simulink model "PID"  (R2024b)
settings: Solver=VariableStepAuto  StartTime=0.0  StopTime=200  FixedStep=1e-3  RelTol=1e-3
undefined symbols (not defined in the file): Orientation, Position
libraries: robotlib x3, simulink_extras x3, sharedutil x2
settings Model: SimulationMode=accelerator  Creator=cdsouza  LastModifiedBy=조홍민
settings SolverCC: ZeroCrossAlgorithm=Adaptive  AlgebraicLoopSolver=TrustRegion
settings DataIOCC: ReturnWorkspaceOutputs=off
settings OptimizationCC: EnhancedBackFolding=on  PassReuseOutputArgsAs=Individual arguments  ZeroExternalMemoryAtStartup=off  ZeroInternalMemoryAtStartup=off  MaxStackSize=64  OptimizeBlockOrder=speed  DifferentSizesBufferReuse=on  EfficientTunableParamExpr=on
settings DebuggingCC: IgnoredZcDiagnostic=none  ParameterTunabilityLossMsg=error  UnconnectedInputMsg=warning  UnconnectedOutputMsg=warning  UnconnectedLineMsg=warning  ArithmeticOperatorsInVariantConditions=warning
settings HardwareCC: ProdBitPerPointer=32  ProdBitPerSizeT=32  ProdBitPerPtrDiffT=32  ProdLargestAtomicFloat=None  ProdIntDivRoundTo=Undefined  ProdEndianess=Unspecified  ProdWordSize=32  ProdHWDeviceType=Generic->Unspecified (assume 32-bit Generic)
settings ModelReferenceCC: EnableRefExpFcnMdlSchedulingChecks=on
settings SFSimCC: MATLABDynamicMemAlloc=off  CustomCodeUndefinedFunction=UseInterfaceOnly
settings RTWCC: Description=Embedded Coder  SystemTargetFile=ert.tlc  HardwareBoard=Robot Operating System (ROS)  TLCOptions="-aInlineSetEventsForThisBaseRateFcn=TLC_FALSE -aSuppressMultiTaskScheduler=TLC_FALSE  -aRateBasedStepFcn=0"  TemplateMakefile=ert_default_tmf  Toolchain=Catkin  TargetLang=C++  GPUComputeCapability=3.5
settings CodeAppCC: ForceParamTrailComments=on  IgnoreCustomStorageClasses=off  OperatorAnnotations=on  SimulinkDataObjDesc=on  SFDataObjDesc=on  InsertBlockDesc=on
settings ERTTargetCC: InlinedParameterPlacement=Hierarchical  DynamicArrayContainerType=coder::array

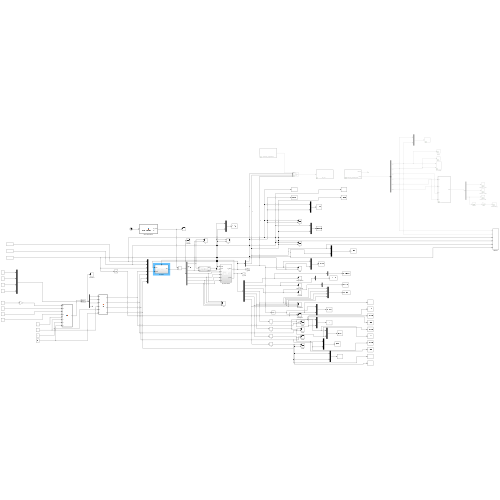
[thumbnail: Simulink's stored preview of the top-level diagram]
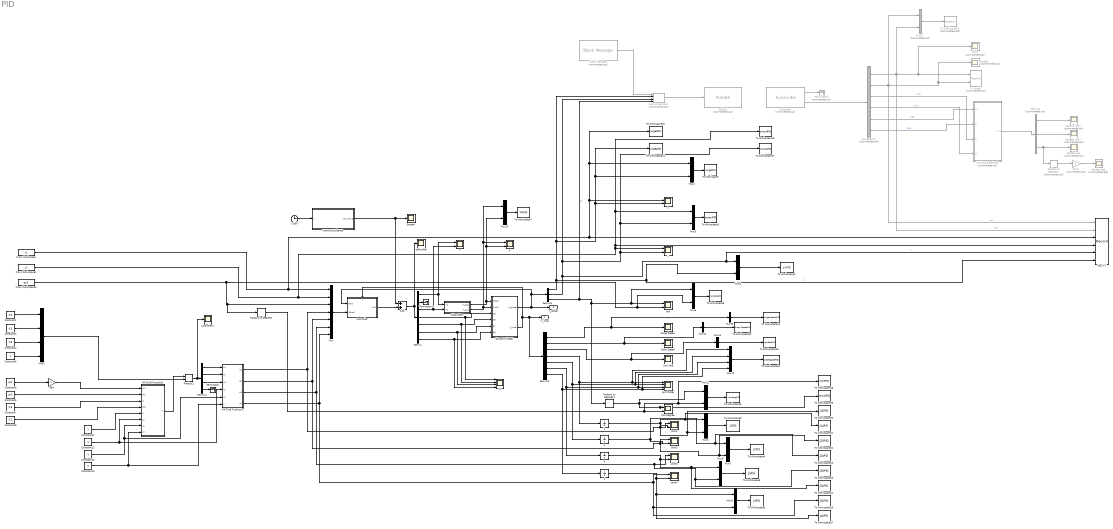
== system PID ==
  {1..4} (4 alike) : Integrator
  Add : Sum
  Blank Message : robotlib/Blank Message  Commented=on  messageClass=Message  entityType=geometry_msgs/Pose  messageType=geometry_msgs/Pose  SampleTime=inf  legacyBusStruct=off
  Bus Assignment : BusAssignment  Commented=on  AssignedSignals=Position.X,Position.Y,Orientation.W
  Bus Selector : BusSelector  Commented=on  OutputSignals=Pose.Position.X,Pose.Position.Y,Pose.Orientation.X,Pose.Orientation.Y,Pose.Orientation.Z,Pose.Orientation.W
  Clock : Clock
  Constant10 : Constant  Value=0
  Constant{5,11..13} (4 alike) : Constant
  Constant2 : Constant  Value=0.5
  Constant3 : Constant  Value=0.3
  Constant4 : Constant  Value=0.8
  Constant6 : Constant  Value=pi/2
  Constant7 : Constant  Value=0.8
  Constant8 : Constant  Value=0.1
  Constant9 : Constant  Value=pi/2
  Controller : Subsystem
      settings: PortSchema="{\"entries\":[{\"content\":{\"sides\":[{\"content\":{\"connectorIds\":[\"In1\",\"In2\"]},\"type\":\"ConnectorPlacement.EquallySpacedRectSide\",\"uuid\":\"f517b411-9821-46d6-bcef-391f15feb496\"},{\"content\":{\"connectorIds\":[\"Out1\"],\"side\":\"RIGHT\"},\"type\":\"ConnectorPlacement.EquallySpacedRectSide\",\"uuid\":\"a797da20-53d3-4f53-a227-0b692005ff54\"},{\"content\":{\"connectorIds\":[\"In3\"],\"side\":\"TOP\"},\"type\":\"ConnectorPlacement.EquallySpacedRectSide\",\"uuid\":\"903174f2-a3c8-433f-ada5-9a38ae3ff1a6\"}]},\"type\":\"ConnectorPlacement.EquallySpacedConnector\",\"uuid\":\"4f0bdd0a-4061-45a8-b959-2bbfa8de12fe\"}],\"packageUris\":[\"http://schema.mathworks.com/mf0/Connector/R2020b\"],\"version\":\"1.0\"}"
  Demux : Demux  Outputs=7
  Demux1 : Demux
  Demux2 : Demux  Outputs=3
  Demux3 : Demux  Outputs=7
  Demux4 : Demux  Commented=on  Outputs=3
  Dynamic Model : Subsystem
  FT : Scope  NumInputPorts=4
  From Workspace : FromWorkspace  VariableName=x1  SampleTime=-1
  From Workspace1 : FromWorkspace  VariableName=y1  SampleTime=-1
  From Workspace2 : FromWorkspace  VariableName=psi1  SampleTime=-1
  Gain : Gain  Gain=-1
  Gain1 : Gain  Commented=on  Gain=-1
  Gazebo Deg : Scope  Commented=on
  Gazebo Yaw : Scope  Commented=on
  Gazebo Yaw1 : Scope  Commented=on
  Gazebo Yaw2 : Scope  Commented=on
  Joint Rates : Scope  NumInputPorts=4
  Joint{1..4} (4 alike) : Scope  NumInputPorts=2
  MATLAB Function1 : MATLAB Function  TreatAsAtomicUnit=on
  MATLAB Function2 : MATLAB Function  TreatAsAtomicUnit=on
  MATLAB Function4 : MATLAB Function  Commented=on  TreatAsAtomicUnit=on
  Mux : Mux  Inputs=7
  Mux1 : Mux
  Mux{2..11} (10 alike) : Mux  Inputs=2
  Mux12 : Mux
  Mux13 : Mux  Inputs=1
  Mux14 : Mux  Inputs=1
  Mux15 : Mux  Inputs=1
  Mux17 : Mux  Commented=on  Inputs=2
  N : Scope  NumInputPorts=2
  NED-XY : Record  FileSettingsInternal="{\"entries\":[{\"content\":{\"excelSettings\":{\"content\":{},\"type\":\"Streamout.ExcelSettings\"}},\"type\":\"Streamout.FileSettingStorage\",\"uuid\":\"\"}],\"packageUris\":[\"http:\\/\\/schema.mathworks.com\\/mf0\\/streamout_blocks\\/R2020a\"],\"version\":\"1.0\"}"  Layout=[1 1]  SignalsInternal="{\"entries\":[{\"content\":{\"signals\":[{\"content\":{\"blockPath\":[],\"dimensions\":[1],\"domain\":\"\",\"lineColor\":\"#a2142f\",\"plots\":[ 1 ],\"port\":1,\"signalID\":1,\"signalName\":\"<Y>\"},\"type\":\"RecordBlkView.Signal\",\"uuid\":\"\"},{\"content\":{\"blockPath\":[],\"dimensions\":[1],\"domain\":\"\",\"lineColor\":\"#139fff\",\"plots\":[ 1 ],\"port\":2,\"signalID\":2,\"signalName\":\"<X>\"},\"type\":\"RecordBlkView.Signal\",\"uuid\":\"\"},{\"content\":{\"blockPath\":[],\"dimensions\":[1],\"domain\":\"\",\"lineColor\":\"#ff6929\",\"plots\":[ 1 ],\"port\":3,\"signalID\":3,\"signalName\":\"From\\nWorkspace\"},\"type\":\"RecordBlkView.Signal\",\"uuid\":\"\"},{\"content\":{\"blockPath\":[],\"dimensions\":[1],\"domain\":\"\",\"lineColor\":\"#b746ff\",\"plots\":[ 1 ],\"port\":4,\"signalID\":4,\"signalName\":\"From\\nWorkspace1\"},\"type\":\"RecordBlkView.Signal\",\"uuid\":\"\"},{\"content\":{\"blockPath\":[],\"dimensions\":[1],\"domain\":\"\",\"lineColor\":\"#139fff\",\"plots\":[ 1 ],\"port\":5,\"signalID\":5,\"signalName\":\"Y\"},\"type\":\"RecordBlkView.Signal\",\"uuid\":\"\"},{\"content\":{\"blockPath\":[],\"dimensions\":[1],\"domain\":\"\",\"lineColor\":\"#ff6929\",\"plots\":[ 1 ],\"port\":6,\"signalID\":6,\"signalName\":\"X\"},\"type\":\"RecordBlkView.Signal\",\"uuid\":\"\"}]},\"type\":\"RecordBlkView.InputSignals\",\"uuid\":\"\"}],\"packageUris\":[\"http:\\/\\/schema.mathworks.com\\/mf0\\/streamout_blocks\\/R2020a\"],\"version\":\"1.0\"}"  VisualizationBindings="{\"xyplotplugin\":{\"info\":[{\"series\":[{\"bindingParametersList\":[{\"parameter\":\"X-Axis\",\"signalID\":1,\"signalName\":\"<Y>\"},{\"parameter\":\"Y-Axis\",\"signalID\":2,\"signalName\":\"<X>\"}],\"seriesID\":0},{\"bindingParametersList\":[{\"parameter\":\"X-Axis\",\"signalID\":4,\"signalName\":\"From\\nWorkspace1\"},{\"parameter\":\"Y-Axis\",\"signalID\":3,\"signalName\":\"From\\nWorkspace\"}],\"seriesID\":1},{\"bindingParametersList\":[{\"parameter\":\"X-Axis\",\"signalID\":5,\"signalName\":\"Y\"},{\"parameter\":\"Y-Axis\",\"signalID\":6,\"signalName\":\"X\"}],\"seriesID\":2}],\"subplotID\":1}]}}"  CompatibilityTag=XY  st=-1
  Product2 : Product  Multiplication=Matrix(*)
  Publish : robotlib/Publish  Commented=on  topicSource=Specify your own  topic=/to_ros  messageType=geometry_msgs/Pose  legacyBusStruct=off  messageQueueLength=1
  Radians to Degrees : simulink_extras/Transformations/Radians to Degrees
  Radians to Degrees1 : simulink_extras/Transformations/Radians to Degrees
  Radians to Degrees2 : simulink_extras/Transformations/Radians to Degrees  Commented=on
  Scope4 : Scope
  Scope5 : Scope  Commented=on
  Subscribe : robotlib/Subscribe  Commented=on  topicSource=Select from ROS network  topic=/mavros/local_position/pose  messageType=geometry_msgs/PoseStamped  SampleTime=-1  legacyBusStruct=off  messageQueueLength=1
  Subsystem : Subsystem
  Surge Speed : Scope
  Sway Speed : Scope
  T : Scope  NumInputPorts=2
  Terminator : Terminator
  Terminator2 : Terminator
  Terminator3 : Terminator  Commented=on
  To Workspace : ToWorkspace  VariableName=surgePID  SampleTime=-1
      settings: Save2DSignal=2-D array (concatenate along first dimension)
  To Workspace1 : ToWorkspace  VariableName=swayPID  SampleTime=-1
      settings: Save2DSignal=2-D array (concatenate along first dimension)
  To Workspace10 : ToWorkspace  VariableName=JointRatesPID  SampleTime=-1
      settings: Save2DSignal=2-D array (concatenate along first dimension)
  To Workspace11 : ToWorkspace  VariableName=SurgeSpeedPID  SampleTime=-1
      settings: Save2DSignal=2-D array (concatenate along first dimension)
  To Workspace12 : ToWorkspace  VariableName=SwaySpeedPID  SampleTime=-1
      settings: Save2DSignal=2-D array (concatenate along first dimension)
  To Workspace13 : ToWorkspace  VariableName=YawRatePID  SampleTime=-1
      settings: Save2DSignal=2-D array (concatenate along first dimension)
  To Workspace14 : ToWorkspace  VariableName=surgeaPID  SampleTime=-1
      settings: Save2DSignal=2-D array (concatenate along first dimension)
  To Workspace15 : ToWorkspace  VariableName=surgedPID  SampleTime=-1
      settings: Save2DSignal=2-D array (concatenate along first dimension)
  To Workspace16 : ToWorkspace  VariableName=swaydPID  SampleTime=-1
      settings: Save2DSignal=2-D array (concatenate along first dimension)
  To Workspace17 : ToWorkspace  VariableName=swayaPID  SampleTime=-1
      settings: Save2DSignal=2-D array (concatenate along first dimension)
  To Workspace18 : ToWorkspace  VariableName=YawDPID  SampleTime=-1
      settings: Save2DSignal=2-D array (concatenate along first dimension)
  To Workspace19 : ToWorkspace  VariableName=YawAPID  SampleTime=-1
      settings: Save2DSignal=2-D array (concatenate along first dimension)
  To Workspace2 : ToWorkspace  VariableName=yxPID  SampleTime=-1
  To Workspace20 : ToWorkspace  VariableName=J1DPID  SampleTime=-1
      settings: Save2DSignal=2-D array (concatenate along first dimension)
  To Workspace21 : ToWorkspace  VariableName=J1APID  SampleTime=-1
      settings: Save2DSignal=2-D array (concatenate along first dimension)
  To Workspace22 : ToWorkspace  VariableName=J2DPID  SampleTime=-1
      settings: Save2DSignal=2-D array (concatenate along first dimension)
  To Workspace23 : ToWorkspace  VariableName=J2APID  SampleTime=-1
      settings: Save2DSignal=2-D array (concatenate along first dimension)
  To Workspace24 : ToWorkspace  VariableName=J3APID  SampleTime=-1
      settings: Save2DSignal=2-D array (concatenate along first dimension)
  To Workspace25 : ToWorkspace  VariableName=J3DPID  SampleTime=-1
      settings: Save2DSignal=2-D array (concatenate along first dimension)
  To Workspace26 : ToWorkspace  VariableName=J4DPID  SampleTime=-1
      settings: Save2DSignal=2-D array (concatenate along first dimension)
  To Workspace27 : ToWorkspace  VariableName=J4APID  SampleTime=-1
      settings: Save2DSignal=2-D array (concatenate along first dimension)
  To Workspace29 : ToWorkspace  Commented=on  VariableName=Gazeboxy  SampleTime=-1
  To Workspace3 : ToWorkspace  VariableName=J1PID  SampleTime=-1
      settings: Save2DSignal=2-D array (concatenate along first dimension)
  To Workspace4 : ToWorkspace  VariableName=J2PID  SampleTime=-1
      settings: Save2DSignal=2-D array (concatenate along first dimension)
  To Workspace5 : ToWorkspace  VariableName=J3PID  SampleTime=-1
      settings: Save2DSignal=2-D array (concatenate along first dimension)
  To Workspace6 : ToWorkspace  VariableName=J4PID  SampleTime=-1
      settings: Save2DSignal=2-D array (concatenate along first dimension)
  To Workspace7 : ToWorkspace  VariableName=THPID  SampleTime=-1
      settings: Save2DSignal=2-D array (concatenate along first dimension)
  To Workspace8 : ToWorkspace  VariableName=YawDataPID  SampleTime=-1
      settings: Save2DSignal=2-D array (concatenate along first dimension)
  To Workspace9 : ToWorkspace  VariableName=YawDegPID  SampleTime=-1
      settings: Save2DSignal=2-D array (concatenate along first dimension)
  USVx : Scope  Commented=on
  Wave Disturbance : MATLAB Function  TreatAsAtomicUnit=on
  XY Graph : Record  Commented=on  FileSettingsInternal="{\"entries\":[{\"content\":{\"excelSettings\":{\"content\":{},\"type\":\"Streamout.ExcelSettings\"}},\"type\":\"Streamout.FileSettingStorage\",\"uuid\":\"\"}],\"packageUris\":[\"http:\\/\\/schema.mathworks.com\\/mf0\\/streamout_blocks\\/R2020a\"],\"version\":\"1.0\"}"  Layout=[1 1]  SignalsInternal="{\"entries\":[{\"content\":{\"signals\":[{\"content\":{\"blockPath\":[],\"dimensions\":[1],\"domain\":\"\",\"lineColor\":\"#a2142f\",\"plots\":[ 1 ],\"port\":1,\"signalID\":1,\"signalName\":\"<X>\"},\"type\":\"RecordBlkView.Signal\",\"uuid\":\"\"},{\"content\":{\"blockPath\":[],\"dimensions\":[1],\"domain\":\"\",\"lineColor\":\"#139fff\",\"plots\":[ 1 ],\"port\":2,\"signalID\":2,\"signalName\":\"<Y>\"},\"type\":\"RecordBlkView.Signal\",\"uuid\":\"\"}]},\"type\":\"RecordBlkView.InputSignals\",\"uuid\":\"\"}],\"packageUris\":[\"http:\\/\\/schema.mathworks.com\\/mf0\\/streamout_blocks\\/R2020a\"],\"version\":\"1.0\"}"  VisualizationBindings="{\"xyplotplugin\":{\"info\":[{\"series\":[{\"bindingParametersList\":[{\"parameter\":\"X-Axis\",\"signalID\":1,\"signalName\":\"<X>\"},{\"parameter\":\"Y-Axis\",\"signalID\":2,\"signalName\":\"<Y>\"}],\"seriesID\":0}],\"subplotID\":1}]}}"  CompatibilityTag=XY
  Y : Scope  NumInputPorts=2
  Yaw : Scope  NumInputPorts=2
  Yaw Degree : Scope  NumInputPorts=2
  Yaw rate : Scope
  controller : Scope
  controller1 : Scope
  x : Scope  NumInputPorts=2
  V_local : Outport  VectorParamsAs1DForOutWhenUnconnected=off
  n_global : Outport  Port=2  VectorParamsAs1DForOutWhenUnconnected=off
  wires:
  Subsystem/1(T_stbd) -> Mux10/2, N/2, Dynamic Model/1(Tstbd)
  Subsystem/2(T_port) -> Mux10/1, N/1, Dynamic Model/2(Tport)
  Dynamic Model/1(n_global) -> Controller/1(Etha), Demux2/1, n_global/1
  Demux3/1 -> Mux15/1, Surge Speed/1
  Demux3/3 -> Mux14/1, Yaw rate/1
  Dynamic Model/2(V_local) -> Controller/3(v), V_local/1, Demux3/1
  Demux3/2 -> Mux13/1, Sway Speed/1
  Demux/1 -> T/1, Subsystem/1(Tx)
  Demux/2 -> Terminator2/1
  Demux/3 -> Subsystem/2(Tz), T/2
  Add/1 -> Demux/1, controller/1
  From Workspace/1 -> To Workspace15/1, Mux2/1, x/1, NED-XY/3, Mux/1
  From Workspace1/1 -> Mux3/1, To Workspace16/1, NED-XY/4, Y/1, Mux/2
  Mux/1 -> Controller/2(Ethad)
  MATLAB Function2/1(q1) -> Mux/4, Joint1/1, To Workspace20/1, Mux6/2
  MATLAB Function2/2(q2) -> Mux/5, Joint2/1, To Workspace22/1, Mux7/2
  MATLAB Function2/3(q3) -> Mux/6, Joint3/1, To Workspace25/1, Mux8/2
  MATLAB Function2/4(q4) -> Mux/7, Joint4/1, To Workspace26/1, Mux9/2
  Demux/4 -> FT/1, Dynamic Model/3(q5)
  Demux/5 -> FT/2, Dynamic Model/4(q6)
  Demux/6 -> FT/3, Dynamic Model/5(q7)
  Demux/7 -> FT/4, Dynamic Model/6(q8)
  Demux3/4 -> 1/1, Joint Rates/1, Mux12/1
  Demux3/5 -> 2/1, Joint Rates/2, Mux12/2
  Demux3/6 -> 3/1, Joint Rates/3, Mux12/3
  Demux3/7 -> Joint Rates/4, Mux12/4, 4/1
  Radians to Degrees1/1 -> To Workspace19/1, Yaw Degree/1, Mux11/1
  Radians to Degrees/1 -> Mux11/2, To Workspace18/1, Yaw Degree/2
  1/1 -> Joint1/2, To Workspace21/1, Mux6/1
  2/1 -> Joint2/2, To Workspace23/1, Mux7/1
  3/1 -> Joint3/2, To Workspace24/1, Mux8/1
  4/1 -> Joint4/2, To Workspace27/1, Mux9/1
  Mux2/1 -> To Workspace/1
  Mux3/1 -> To Workspace1/1
  Mux5/1 -> To Workspace8/1
  Mux4/1 -> To Workspace2/1
  Mux6/1 -> To Workspace3/1
  Mux7/1 -> To Workspace4/1
  Mux8/1 -> To Workspace5/1
  Mux9/1 -> To Workspace6/1
  Mux10/1 -> To Workspace7/1
  Constant8/1 -> MATLAB Function1/4(th3)
  Demux1/4 -> Terminator/1
  Constant3/1 -> Mux1/2
  Mux1/1 -> Product2/2
  Constant9/1 -> Gain/1
  Constant2/1 -> Mux1/1
  Constant7/1 -> MATLAB Function1/3(d)
  Constant13/1 -> MATLAB Function1/7(L2), MATLAB Function2/5(L2)
  Constant10/1 -> MATLAB Function1/8(L3), MATLAB Function2/6(h)
  Constant6/1 -> MATLAB Function1/2(th2)
  Gain/1 -> MATLAB Function1/1(th1)
  Demux1/1 -> MATLAB Function2/1(Px)
  Constant11/1 -> MATLAB Function1/5(h)
  Demux1/3 -> MATLAB Function2/3(Pz)
  Constant4/1 -> Mux1/3
  Demux1/2 -> MATLAB Function2/2(Py)
  Product2/1 -> controller1/1, Demux1/1
  Constant12/1 -> MATLAB Function1/6(L1), MATLAB Function2/4(L1)
  Constant5/1 -> Mux1/4
  MATLAB Function1/1(T) -> Product2/1
  Mux11/1 -> To Workspace9/1
  Mux12/1 -> To Workspace10/1
  Mux13/1 -> To Workspace12/1
  Mux14/1 -> To Workspace13/1
  Mux15/1 -> To Workspace11/1
  From Workspace2/1 -> Yaw/2, Mux5/2, Radians to Degrees/1, Mux/3
  Demux2/3 -> Radians to Degrees1/1, Yaw/1, Mux5/1, Bus Assignment/4  "Z"
  Demux2/1 -> Bus Assignment/2, To Workspace14/1, Mux2/2, x/2, Mux4/2, NED-XY/6  "X"
  Bus Assignment/1 -> Publish/1
  Blank Message/1 -> Bus Assignment/1
  Demux2/2 -> Bus Assignment/3, Y/2, Mux3/2, To Workspace17/1, NED-XY/5, Mux4/1  "Y"
  Bus Selector/4 -> MATLAB Function4/4(qz)  "<Y>"
  Demux4/1 -> Gazebo Yaw1/1
  Bus Selector/6 -> MATLAB Function4/2(qx)  "<W>"
  Bus Selector/1 -> NED-XY/2, Mux17/2, XY Graph/1, USVx/1  "<X>"
  Bus Selector/5 -> MATLAB Function4/1(qw)  "<Z>"
  Bus Selector/2 -> NED-XY/1, Mux17/1, Scope5/1, XY Graph/2  "<Y>"
  Subscribe/1 -> Terminator3/1
  Radians to Degrees2/1 -> Gain1/1
  Demux4/3 -> Gazebo Yaw/1, Radians to Degrees2/1
  Mux17/1 -> To Workspace29/1
  Bus Selector/3 -> MATLAB Function4/3(qy)  "<X>"
  Gain1/1 -> Gazebo Deg/1
  Demux4/2 -> Gazebo Yaw2/1
  MATLAB Function4/1(XYZ) -> Demux4/1
  Subscribe/2 -> Bus Selector/1
  Clock/1 -> Wave Disturbance/1(t)
  Wave Disturbance/1(tau_wave) -> Add/1, Scope4/1
  Controller/1(Out) -> Add/2

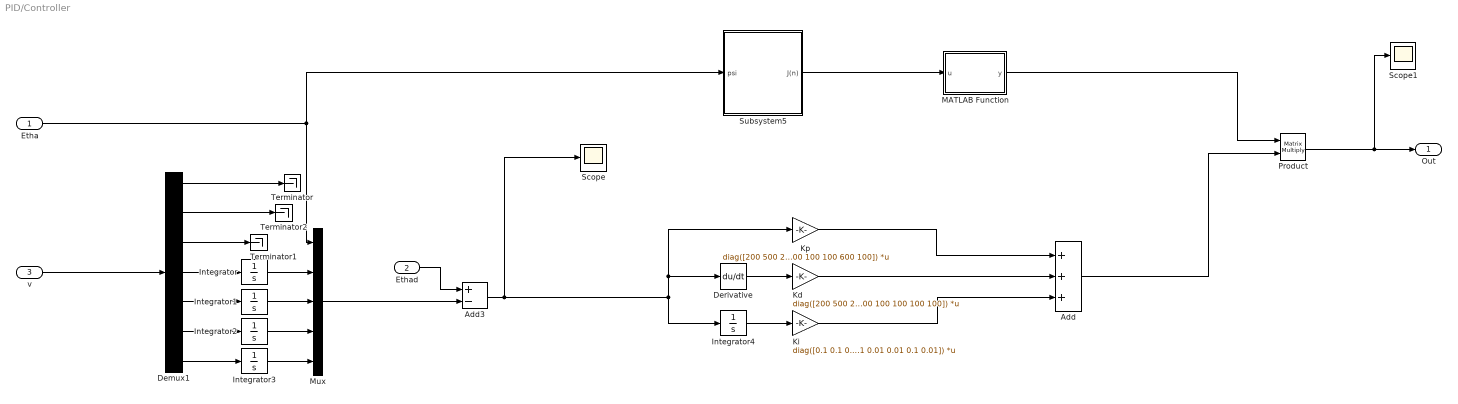
== system PID/Controller ==
  Etha : Inport
  Ethad : Inport  Port=2
  v : Inport  Port=3
  Add : Sum  Inputs=+++
  Add3 : Sum  Inputs=+-
  Demux1 : Demux  Outputs=7
  Derivative : Derivative
  Integrator{,1..4} (5 alike) : Integrator
  Kd : Gain  Gain=diag([200 500 200 100 100 100 100])  Multiplication=Matrix(K*u)
  Ki : Gain  Gain=diag([0.1 0.1 0.1 0.01 0.01 0.1 0.01])  Multiplication=Matrix(K*u)
  Kp : Gain  Gain=diag([200 500 200 100 100 600 100])  Multiplication=Matrix(K*u)
  MATLAB Function : MATLAB Function  TreatAsAtomicUnit=on
  Mux : Mux  Inputs=5
  Product : Product  Multiplication=Matrix(*)
  Scope : Scope
  Scope1 : Scope
  Subsystem5 : Subsystem
  Terminator : Terminator
  Terminator1 : Terminator
  Terminator2 : Terminator
  Out : Outport
  wires:
  Ethad/1 -> Add3/1
  v/1 -> Demux1/1
  Integrator3/1 -> Mux/5
  Integrator2/1 -> Mux/4
  Demux1/7 -> Integrator3/1
  Demux1/5 -> Integrator1/1
  Demux1/6 -> Integrator2/1
  Demux1/2 -> Terminator2/1
  Demux1/3 -> Terminator1/1
  Integrator/1 -> Mux/2
  Integrator1/1 -> Mux/3
  Demux1/1 -> Terminator/1
  Demux1/4 -> Integrator/1
  Etha/1 -> Subsystem5/1(psi), Mux/1
  Mux/1 -> Add3/2
  Add3/1 -> Derivative/1, Kp/1, Integrator4/1, Scope/1
  Subsystem5/1(J(n)) -> MATLAB Function/1(u)
  Add/1 -> Product/2
  MATLAB Function/1(y) -> Product/1
  Product/1 -> Scope1/1, Out/1
  Derivative/1 -> Kd/1
  Kp/1 -> Add/1
  Kd/1 -> Add/2
  Integrator4/1 -> Ki/1
  Ki/1 -> Add/3

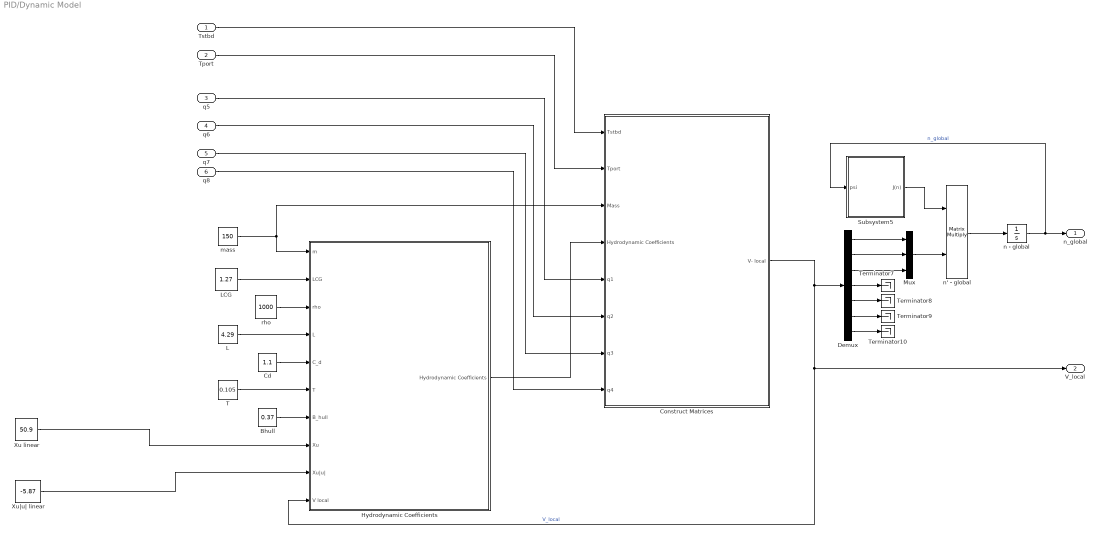
== system PID/Dynamic Model ==
  Tstbd : Inport
  Tport : Inport  Port=2
  q5 : Inport  Port=3
  q6 : Inport  Port=4
  q7 : Inport  Port=5
  q8 : Inport  Port=6
  "Bhull " : Constant  Value=0.37
  Cd : Constant  Value=1.1
  Construct Matrices : Subsystem
  Demux : Demux  Outputs=7
  Hydrodynamic Coefficients : Subsystem
  L : Constant  Value=4.29
  LCG : Constant  Value=1.27
  Mux : Mux  Inputs=3
  Subsystem5 : Subsystem
  T : Constant  Value=0.105
  Terminator{7..10} (4 alike) : Terminator
  Xu linear : Constant  Value=50.9
  Xu|u| linear : Constant  Value=-5.87
  mass : Constant  Value=150
  n - global : Integrator  InitialCondition=[0 0 0]
  n' - global : Product  Multiplication=Matrix(*)
  rho : Constant  Value=1000
  n_global : Outport  VectorParamsAs1DForOutWhenUnconnected=off
  V_local : Outport  Port=2  VectorParamsAs1DForOutWhenUnconnected=off
  wires:
  n - global/1 -> Subsystem5/1(psi), n_global/1  "n_global"
  Cd/1 -> Hydrodynamic Coefficients/5(C_d)
  n' - global/1 -> n - global/1
  Subsystem5/1(J(n)) -> n' - global/1
  rho/1 -> Hydrodynamic Coefficients/3(rho)
  L/1 -> Hydrodynamic Coefficients/4(L)
  Tport/1 -> Construct Matrices/2(Tport)
  Tstbd/1 -> Construct Matrices/1(Tstbd)
  mass/1 -> Hydrodynamic Coefficients/1(m), Construct Matrices/3("Mass ")
  Hydrodynamic Coefficients/1("Hydrodynamic Coefficients ") -> Construct Matrices/4(Hydrodynamic Coefficients)
  T/1 -> Hydrodynamic Coefficients/6(T)
  "Bhull "/1 -> Hydrodynamic Coefficients/7(B_hull)
  Xu|u| linear/1 -> Hydrodynamic Coefficients/9(Xu|u|)
  LCG/1 -> Hydrodynamic Coefficients/2(LCG)
  Xu linear/1 -> Hydrodynamic Coefficients/8(Xu)
  q8/1 -> Construct Matrices/8(q4)
  q7/1 -> Construct Matrices/7(q3)
  q5/1 -> Construct Matrices/5(q1)
  q6/1 -> Construct Matrices/6(q2)
  Demux/1 -> Mux/1
  Demux/3 -> Mux/3
  Mux/1 -> n' - global/2
  Demux/7 -> Terminator10/1
  Demux/4 -> Terminator7/1
  Demux/2 -> Mux/2
  Demux/6 -> Terminator9/1
  Demux/5 -> Terminator8/1
  Construct Matrices/1(V- local) -> Demux/1, Hydrodynamic Coefficients/10(V local), V_local/1  "V_local"

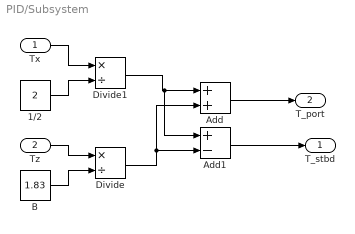
== system PID/Subsystem ==
  Tx : Inport
  Tz : Inport  Port=2
  1/2 : Constant  Value=2
  Add : Sum
  Add1 : Sum  Inputs=+-
  B : Constant  Value=1.83
  Divide : Product  Inputs=*/
  Divide1 : Product  Inputs=*/
  T_stbd : Outport
  T_port : Outport  Port=2
  wires:
  Tz/1 -> Divide/1
  B/1 -> Divide/2
  Tx/1 -> Divide1/1
  1/2/1 -> Divide1/2
  Divide1/1 -> Add1/1, Add/1
  Divide/1 -> Add1/2, Add/2
  Add/1 -> T_port/1
  Add1/1 -> T_stbd/1

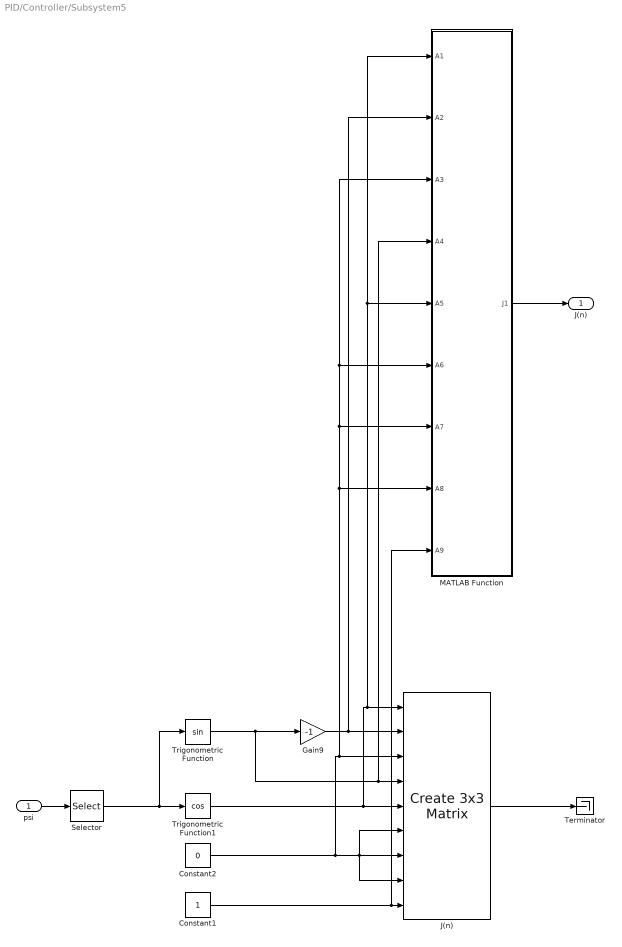
== system PID/Controller/Subsystem5 ==
  psi : Inport
  " J(n)" : sharedutil/Create 3x3 Matrix  aMode=aMode
  Constant1 : Constant
  Constant2 : Constant  Value=0
  Gain9 : Gain  Gain=-1
  MATLAB Function : MATLAB Function  TreatAsAtomicUnit=on
  Selector : Selector  InputPortWidth=3  IndexOptions=Index vector (dialog)  Indices=3  OutputSizes=1
  Terminator : Terminator
  Trigonometric Function : Trigonometry
  Trigonometric Function1 : Trigonometry  Operator=cos
  J(n) : Outport
  wires:
  " J(n)"/1 -> Terminator/1
  Constant1/1 -> MATLAB Function/9(A9), " J(n)"/9
  Trigonometric Function1/1 -> " J(n)"/5, " J(n)"/1, MATLAB Function/1(A1), MATLAB Function/5(A5)
  psi/1 -> Selector/1
  Trigonometric Function/1 -> MATLAB Function/4(A4), " J(n)"/4, Gain9/1
  Selector/1 -> Trigonometric Function1/1, Trigonometric Function/1
  Constant2/1 -> " J(n)"/8, " J(n)"/7, " J(n)"/6, MATLAB Function/8(A8), MATLAB Function/3(A3), MATLAB Function/6(A6), MATLAB Function/7(A7), " J(n)"/3
  Gain9/1 -> " J(n)"/2, MATLAB Function/2(A2)
  MATLAB Function/1(J1) -> J(n)/1

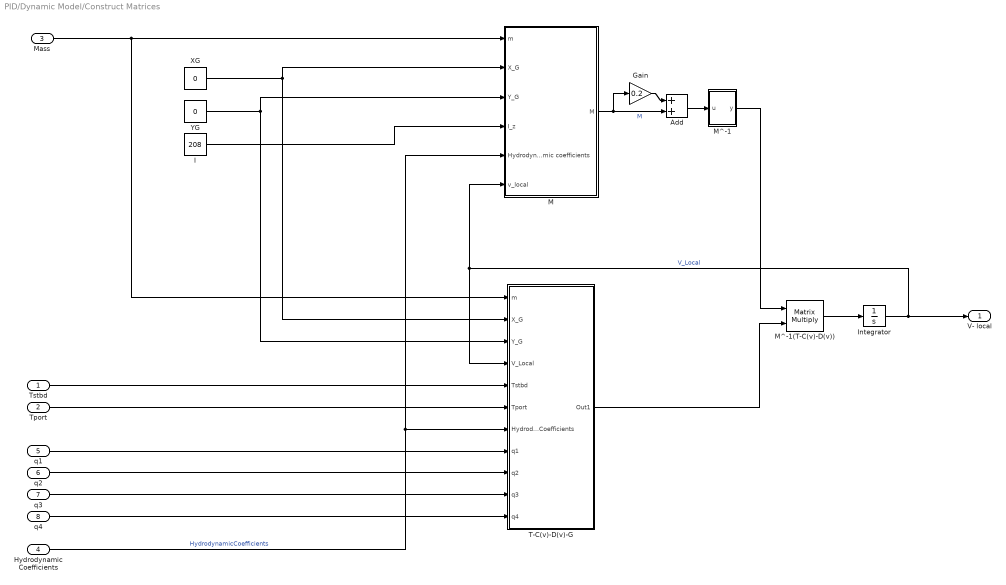
== system PID/Dynamic Model/Construct Matrices ==
  Tstbd : Inport
  Tport : Inport  Port=2
  "Mass " : Inport  Port=3
  Hydrodynamic Coefficients : Inport  Port=4
  q1 : Inport  Port=5
  q2 : Inport  Port=6
  q3 : Inport  Port=7
  q4 : Inport  Port=8
  Add : Sum
  Gain : Gain  Gain=0.2
  I : Constant  Value=208
  Integrator : Integrator
  M : Subsystem
  M^-1 : MATLAB Function  TreatAsAtomicUnit=on
  M^-1(T-C(v)-D(v)) : Product  Multiplication=Matrix(*)
  T-C(v)-D(v)-G : Subsystem
  XG : Constant  Value=0
  YG : Constant  Value=0
  V- local : Outport  VectorParamsAs1DForOutWhenUnconnected=off
  wires:
  M/1(M) -> Gain/1, Add/2  "M"
  Integrator/1 -> V- local/1, M/6(v_local), T-C(v)-D(v)-G/4(V_Local)  "V_Local"
  M^-1(T-C(v)-D(v))/1 -> Integrator/1
  I/1 -> M/4(I_z)
  M^-1/1(y) -> M^-1(T-C(v)-D(v))/1
  Hydrodynamic Coefficients/1 -> M/5(Hydrodynamic coefficients), T-C(v)-D(v)-G/7(HydrodynamicCoefficients)  "HydrodynamicCoefficients"
  YG/1 -> M/3(Y_G), T-C(v)-D(v)-G/3(Y_G)
  "Mass "/1 -> T-C(v)-D(v)-G/1(m), M/1(m)
  XG/1 -> M/2(X_G), T-C(v)-D(v)-G/2(X_G)
  Tstbd/1 -> T-C(v)-D(v)-G/5(Tstbd)
  Tport/1 -> T-C(v)-D(v)-G/6(Tport)
  T-C(v)-D(v)-G/1(Out1) -> M^-1(T-C(v)-D(v))/2
  q3/1 -> T-C(v)-D(v)-G/10(q3)
  q1/1 -> T-C(v)-D(v)-G/8(q1)
  q4/1 -> T-C(v)-D(v)-G/11(q4)
  q2/1 -> T-C(v)-D(v)-G/9(q2)
  Add/1 -> M^-1/1(u)
  Gain/1 -> Add/1

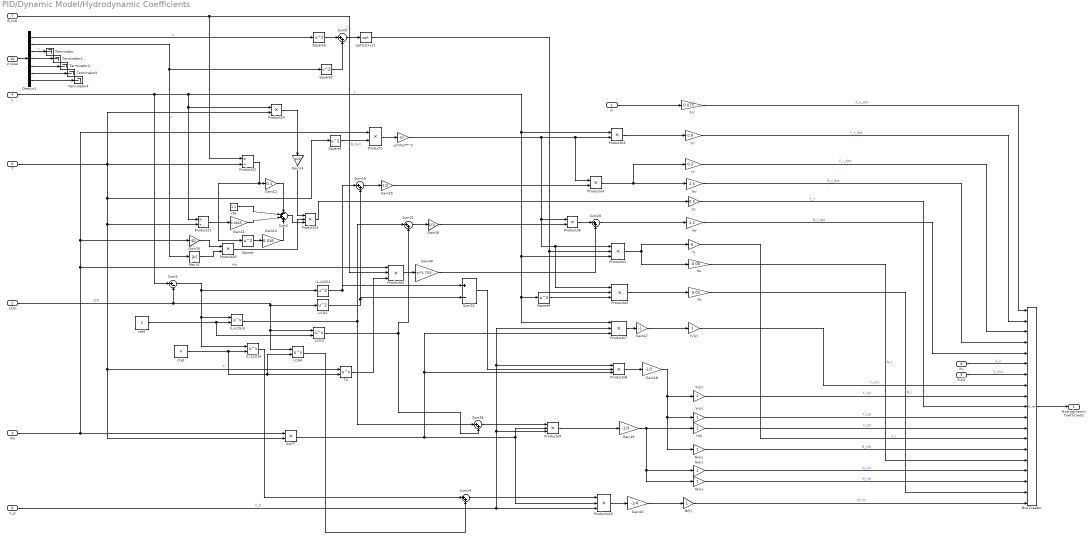
== system PID/Dynamic Model/Hydrodynamic Coefficients ==
  m : Inport
  LCG : Inport  Port=2
  rho : Inport  Port=3
  L : Inport  Port=4
  C_d : Inport  Port=5
  T : Inport  Port=6
  B_hull : Inport  Port=7
  Xu : Inport  Port=8
  Xu|u| : Inport  Port=9
  V local : Inport  Port=10
  (L-LCG)2 : Math  Operator=square  SignedPower=on
  (L-LCG)3 : Math  Operator=pow  SignedPower=on
  (L-LCG)4 : Math  Operator=pow  SignedPower=on
  -pi*rho*T^2 : Gain  Gain=-pi
  Abs v1 : Abs  SaturateOnIntegerOverflow=off
  Bus Creator : BusCreator  Inputs=19
  Demux1 : Demux  Outputs=7
  Gain10 : Gain  Gain=-40
  Gain11 : Gain  Gain=0.0045
  Gain12 : Gain  Gain=0.1
  Gain13 : Gain  Gain=0.016
  Gain14 : Gain  Gain=pi/2
  Gain15 : Gain  Gain=1/2
  Gain16 : Gain  Gain=1/3
  Gain17 : Gain  Gain=-1
  Gain18 : Gain  Gain=-1/2
  Gain19 : Gain  Gain=-1/3
  Gain20 : Gain  Gain=-1/4
  Gain40 : Gain  Gain=-pi*4.75/4
  LCG2 : Math  Operator=square  SignedPower=on
  LCG3 : Math  Operator=pow  SignedPower=on
  LCG4 : Math  Operator=pow  SignedPower=on
  Nr : Gain  Gain=0.02
  Nr' : Gain  Gain=1.2
  Nr|r| : Gain
  Nr|v| : Gain
  Nv : Gain  Gain=0.06
  Nv' : Gain  Gain=2.5
  Nv|r| : Gain
  Nv|v| : Gain
  Product20 : Product
  Product21 : Product  Inputs=*/
  Product22 : Product  Inputs=*/
  Product23 : Product  Inputs=3
  Product24 : Product
  Producto{,3..4,6} (4 alike) : Product
  Producto{1..2,5,7..10} (7 alike) : Product  Inputs=3
  Square{,1..4} (5 alike) : Math  Operator=square  SignedPower=on
  Sum{5,19..21,23..24} (6 alike) : Sum  Inputs=|++
  Sum2 : Sum  Inputs=-+++
  Sum22 : Sum  Inputs=|+-
  Sum9 : Sum  Inputs=|+-
  T4 : Math  Operator=pow  SignedPower=on
  Terminator{,1..4} (5 alike) : Terminator
  Xu' : Gain  Gain=0.075
  Yr : Gain  Gain=6
  Yr' : Gain  Gain=0.2
  Yr|r| : Gain
  Yr|v| : Gain
  Yv : Gain  Gain=0.5
  Yv' : Gain  Gain=0.9
  Yv|r| : Gain
  Yv|v| : Gain
  cte : Constant  Value=1.1
  cte1 : Constant  Value=4
  cte2 : Constant  Value=3
  rho*T : Product
  sqrt(u2+v2) : Sqrt
  "Hydrodynamic Coefficients " : Outport  VectorParamsAs1DForOutWhenUnconnected=off
  wires:
  m/1 -> Xu'/1
  Nv'/1 -> Bus Creator/4  "N_v_dot"
  Xu'/1 -> Bus Creator/1  "X_u_dot"
  Square/1 -> Gain13/1
  Gain14/1 -> Product23/1
  Product24/1 -> Gain14/1
  Sum9/1 -> (L-LCG)3/1, (L-LCG)4/1, (L-LCG)2/1
  Square4/1 -> Producto2/3
  sqrt(u2+v2)/1 -> Producto2/2, Producto1/2
  Product20/1 -> Product23/2
  Gain13/1 -> Sum2/4
  B_hull/1 -> Producto5/2, Product22/1  "B_hull"
  Square2/1 -> Sum5/2
  Sum20/1 -> Nr'/1
  Gain12/1 -> Sum2/1
  Sum21/1 -> Gain16/1
  LCG4/1 -> Sum24/2
  Sum24/1 -> Producto10/1
  (L-LCG)4/1 -> Sum24/1
  Sum2/1 -> Product23/3
  Producto10/1 -> Gain20/1
  (L-LCG)3/1 -> Sum21/1, Sum23/1
  Producto6/1 -> Sum20/1
  Gain19/1 -> Yr|r|/1, Nr|v|/1, Nv|r|/1
  Gain16/1 -> Producto6/2
  Sum22/1 -> Producto8/2
  Producto3/1 -> Yv'/1
  Gain10/1 -> Product20/1
  cte1/1 -> LCG4/2, T4/2, (L-LCG)4/2
  cte2/1 -> (L-LCG)3/2, LCG3/2
  Product23/1 -> Yv/1
  cte/1 -> Sum2/2
  Producto8/1 -> Gain18/1
  Sum23/1 -> Producto9/1
  Gain20/1 -> Nr|r|/1
  Gain18/1 -> Nv|v|/1, Yr|v|/1, Yv|r|/1
  Yr'/1 -> Bus Creator/3  "Y_r_dot"
  Producto7/1 -> Gain17/1
  Producto9/1 -> Gain19/1
  Gain11/1 -> Sum2/3
  Square1/1 -> Producto/2
  Producto2/1 -> Nr/1
  LCG3/1 -> Sum21/2, Sum23/2
  T4/1 -> Producto5/3
  Gain40/1 -> Sum20/2
  Producto4/1 -> Yr'/1, Nv'/1
  Sum19/1 -> Gain15/1
  Square3/1 -> Sum5/1
  Sum5/1 -> sqrt(u2+v2)/1
  rho/1 -> Producto/1, Gain10/1, Producto5/1, rho*T/1  "rho"
  Abs v1/1 -> Product20/2
  Product21/1 -> Gain11/1
  Gain17/1 -> Yv|v|/1
  (L-LCG)2/1 -> Sum19/1, Sum22/1
  Producto1/1 -> Nv/1, Yr/1
  Product22/1 -> Square/1, Gain12/1
  LCG2/1 -> Sum19/2, Sum22/2
  LCG/1 -> Sum9/2, LCG2/1, LCG3/1, LCG4/1  "LCG"
  Producto/1 -> -pi*rho*T^2/1
  -pi*rho*T^2/1 -> Producto4/1, Producto3/2, Producto2/1, Producto1/1, Producto6/1
  Producto5/1 -> Gain40/1
  Gain15/1 -> Producto4/2
  rho*T/1 -> Producto9/2, Producto10/2, Producto7/3, Producto8/3
  T/1 -> Product21/2, rho*T/2, T4/1, Square1/1, Product22/2, Product24/2  "T"
  L/1 -> Producto7/1, Square4/1, Producto1/3, Producto3/1, Product21/1, Product24/1, Sum9/1  "L"
  C_d/1 -> Producto7/2, Producto8/1, Producto9/3, Producto10/3  "C_d"
  Nv/1 -> Bus Creator/15  "N_v"
  Yv|v|/1 -> Bus Creator/8  "Y_v|v|"
  Yr|r|/1 -> Bus Creator/12  "Y_r|r|"
  Yv/1 -> Bus Creator/10  "Y_v"
  Nv|v|/1 -> Bus Creator/14  "N_v|v|"
  Yr|v|/1 -> Bus Creator/11  "Y_r|v|"
  Nv|r|/1 -> Bus Creator/16  "N_v|r|"
  Yr/1 -> Bus Creator/13  "Y_r"
  Nr|r|/1 -> Bus Creator/19  "N_r|r|"
  Nr/1 -> Bus Creator/18  "N_r"
  Xu|u|/1 -> Bus Creator/7  "X_u|u|"
  Yv|r|/1 -> Bus Creator/9  "Y_v|r|"
  Nr|v|/1 -> Bus Creator/17  "N_r|v|"
  Xu/1 -> Bus Creator/6  "X_u"
  Bus Creator/1 -> "Hydrodynamic Coefficients "/1
  Nr'/1 -> Bus Creator/5  "N_r_dot"
  Yv'/1 -> Bus Creator/2  "Y_v_dot"
  Demux1/1 -> Square3/1  "u"
  V local/1 -> Demux1/1
  Demux1/2 -> Abs v1/1, Square2/1  "v"
  Demux1/3 -> Terminator/1  "r"
  Demux1/4 -> Terminator1/1
  Demux1/5 -> Terminator2/1
  Demux1/6 -> Terminator3/1
  Demux1/7 -> Terminator4/1

== system PID/Dynamic Model/Subsystem5 ==
  psi : Inport
  " J(n)" : sharedutil/Create 3x3 Matrix  aMode=aMode
  Constant1 : Constant
  Constant2 : Constant  Value=0
  Gain9 : Gain  Gain=-1
  Selector : Selector  InputPortWidth=3  IndexOptions=Index vector (dialog)  Indices=3  OutputSizes=1
  Trigonometric Function : Trigonometry
  Trigonometric Function1 : Trigonometry  Operator=cos
  J(n) : Outport  VectorParamsAs1DForOutWhenUnconnected=off
  wires:
  Gain9/1 -> " J(n)"/2
  Trigonometric Function1/1 -> " J(n)"/5, " J(n)"/1
  Trigonometric Function/1 -> " J(n)"/4, Gain9/1
  Constant1/1 -> " J(n)"/9
  psi/1 -> Selector/1
  " J(n)"/1 -> J(n)/1
  Constant2/1 -> " J(n)"/8, " J(n)"/7, " J(n)"/6, " J(n)"/3
  Selector/1 -> Trigonometric Function1/1, Trigonometric Function/1

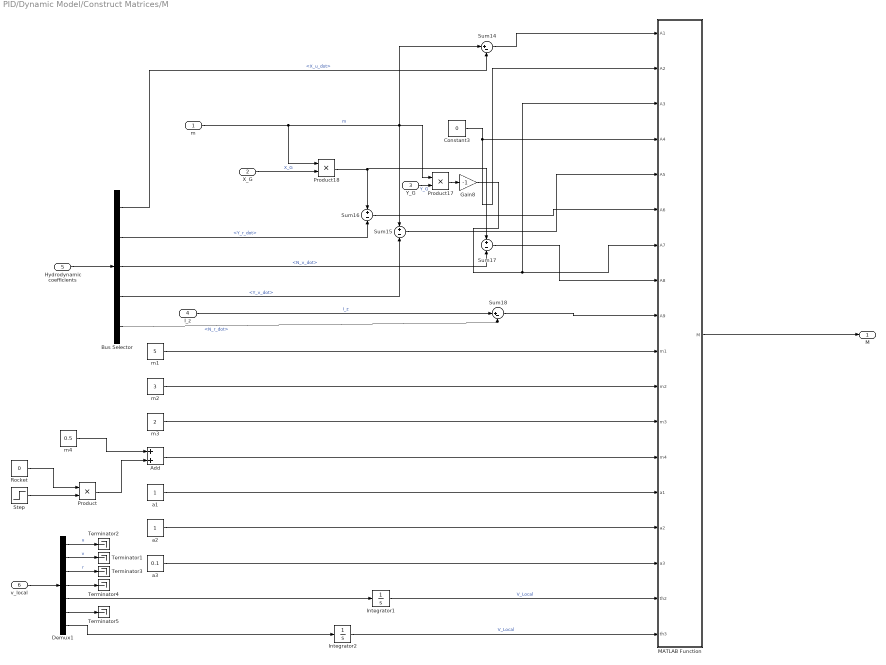
== system PID/Dynamic Model/Construct Matrices/M ==
  m : Inport
  X_G : Inport  Port=2
  Y_G : Inport  Port=3
  I_z : Inport  Port=4
  Hydrodynamic coefficients : Inport  Port=5
  v_local : Inport  Port=6
  Add : Sum
  Bus Selector : BusSelector  OutputSignals=X_u_dot,Y_r_dot,N_v_dot,Y_v_dot,N_r_dot
  Constant3 : Constant  Value=0
  Demux1 : Demux  Outputs=7
  Gain8 : Gain  Gain=-1
  Integrator1 : Integrator
  Integrator2 : Integrator
  MATLAB Function : MATLAB Function  TreatAsAtomicUnit=on
  Product : Product
  Product17 : Product
  Product18 : Product
  Rocket : Constant  Value=0
  Step : Step  Time=40  SampleTime=0
  Sum14 : Sum  Inputs=|+-
  Sum15 : Sum  Inputs=+-
  Sum16 : Sum  Inputs=+-
  Sum17 : Sum  Inputs=+-
  Sum18 : Sum  Inputs=|+-
  Terminator{1..5} (5 alike) : Terminator
  a1 : Constant
  a2 : Constant
  a3 : Constant  Value=0.1
  m1 : Constant  Value=5
  m2 : Constant  Value=3
  m3 : Constant  Value=2
  m4 : Constant  Value=0.5
  M : Outport
  wires:
  Constant3/1 -> MATLAB Function/2(A2), MATLAB Function/4(A4)
  Sum14/1 -> MATLAB Function/1(A1)
  X_G/1 -> Product18/2  "X_G"
  Bus Selector/1 -> Sum14/2  "<X_u_dot>"
  Y_G/1 -> Product17/2  "Y_G"
  Sum18/1 -> MATLAB Function/9(A9)
  Bus Selector/2 -> Sum16/2  "<Y_r_dot>"
  Bus Selector/3 -> Sum17/2  "<N_v_dot>"
  Bus Selector/4 -> Sum15/2  "<Y_v_dot>"
  Sum17/1 -> MATLAB Function/8(A8)
  Sum16/1 -> MATLAB Function/6(A6)
  Bus Selector/5 -> Sum18/2  "<N_r_dot>"
  Sum15/1 -> MATLAB Function/5(A5)
  m/1 -> Sum14/1, Product17/1, Sum15/1, Product18/1  "m"
  MATLAB Function/1(M) -> M/1
  Hydrodynamic coefficients/1 -> Bus Selector/1
  Product17/1 -> Gain8/1
  Gain8/1 -> MATLAB Function/7(A7), MATLAB Function/3(A3)
  I_z/1 -> Sum18/1  "I_z"
  Product18/1 -> Sum17/1, Sum16/1
  m1/1 -> MATLAB Function/10(m1)
  m2/1 -> MATLAB Function/11(m2)
  m3/1 -> MATLAB Function/12(m3)
  m4/1 -> Add/1
  a1/1 -> MATLAB Function/14(a1)
  a2/1 -> MATLAB Function/15(a2)
  a3/1 -> MATLAB Function/16(a3)
  v_local/1 -> Demux1/1
  Demux1/1 -> Terminator2/1  "u"
  Demux1/2 -> Terminator1/1  "v"
  Demux1/3 -> Terminator3/1  "r"
  Demux1/4 -> Terminator4/1
  Demux1/5 -> Integrator1/1
  Demux1/6 -> Terminator5/1
  Demux1/7 -> Integrator2/1
  Integrator1/1 -> MATLAB Function/17(th2)  "V_Local"
  Integrator2/1 -> MATLAB Function/18(th3)  "V_Local"
  Rocket/1 -> Product/1
  Add/1 -> MATLAB Function/13(m4)
  Step/1 -> Product/2
  Product/1 -> Add/2

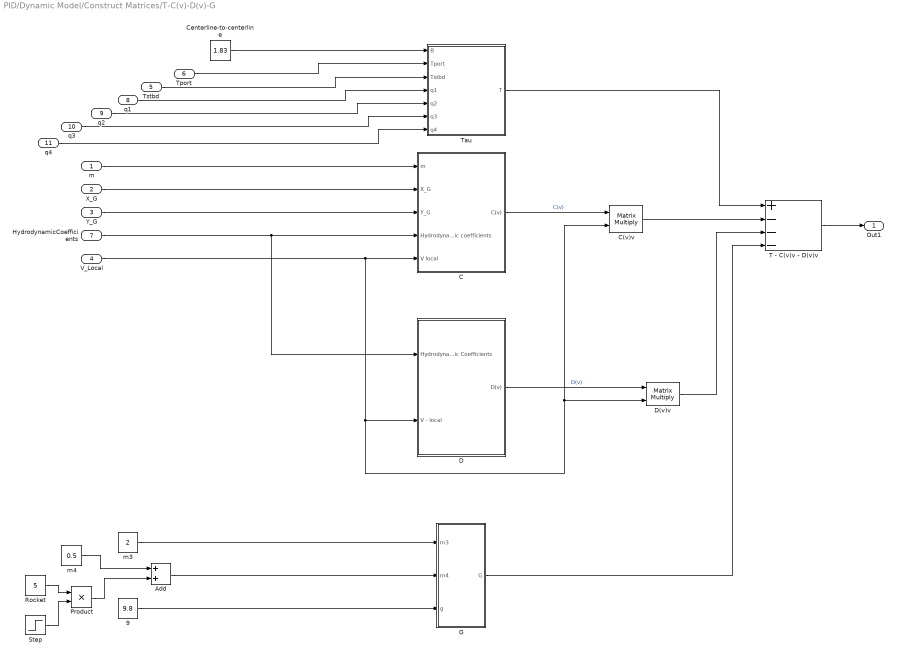
== system PID/Dynamic Model/Construct Matrices/T-C(v)-D(v)-G ==
  m : Inport
  X_G : Inport  Port=2
  Y_G : Inport  Port=3
  V_Local : Inport  Port=4
  Tstbd : Inport  Port=5
  Tport : Inport  Port=6
  HydrodynamicCoefficients : Inport  Port=7
  q1 : Inport  Port=8
  q2 : Inport  Port=9
  q3 : Inport  Port=10
  q4 : Inport  Port=11
  9 : Constant  Value=9.8
  Add : Sum
  C : Subsystem
  C(v)v : Product  Multiplication=Matrix(*)
  Centerline-to-centerline : Constant  Value=1.83
  D : Subsystem
  D(v)v : Product  Multiplication=Matrix(*)
  G : MATLAB Function  TreatAsAtomicUnit=on
  Product : Product
  Rocket : Constant  Value=5
  Step : Step  Time=40  SampleTime=0
  T - C(v)v - D(v)v : Sum  Inputs=+---
  Tau : Subsystem
  m3 : Constant  Value=2
  m4 : Constant  Value=0.5
  Out1 : Outport  VectorParamsAs1DForOutWhenUnconnected=off
  wires:
  V_Local/1 -> C/5(V local), D/2(V - local), D(v)v/2, C(v)v/2
  T - C(v)v - D(v)v/1 -> Out1/1
  D(v)v/1 -> T - C(v)v - D(v)v/3
  C(v)v/1 -> T - C(v)v - D(v)v/2
  Centerline-to-centerline/1 -> Tau/1(B)
  C/1(C(v)) -> C(v)v/1  "C(v)"
  Tau/1(T) -> T - C(v)v - D(v)v/1
  D/1(D(v)) -> D(v)v/1  "D(v)"
  HydrodynamicCoefficients/1 -> D/1(Hydrodynamic Coefficients), C/4(Hydrodynamic coefficients)
  Y_G/1 -> C/3(Y_G)
  X_G/1 -> C/2(X_G)
  m/1 -> C/1(m)
  Tport/1 -> Tau/2(Tport)
  Tstbd/1 -> Tau/3(Tstbd)
  q2/1 -> Tau/5(q2)
  q4/1 -> Tau/7(q4)
  q3/1 -> Tau/6(q3)
  q1/1 -> Tau/4(q1)
  m3/1 -> G/1(m3)
  m4/1 -> Add/1
  9/1 -> G/3(g)
  G/1(G) -> T - C(v)v - D(v)v/4
  Rocket/1 -> Product/1
  Add/1 -> G/2(m4)
  Step/1 -> Product/2
  Product/1 -> Add/2

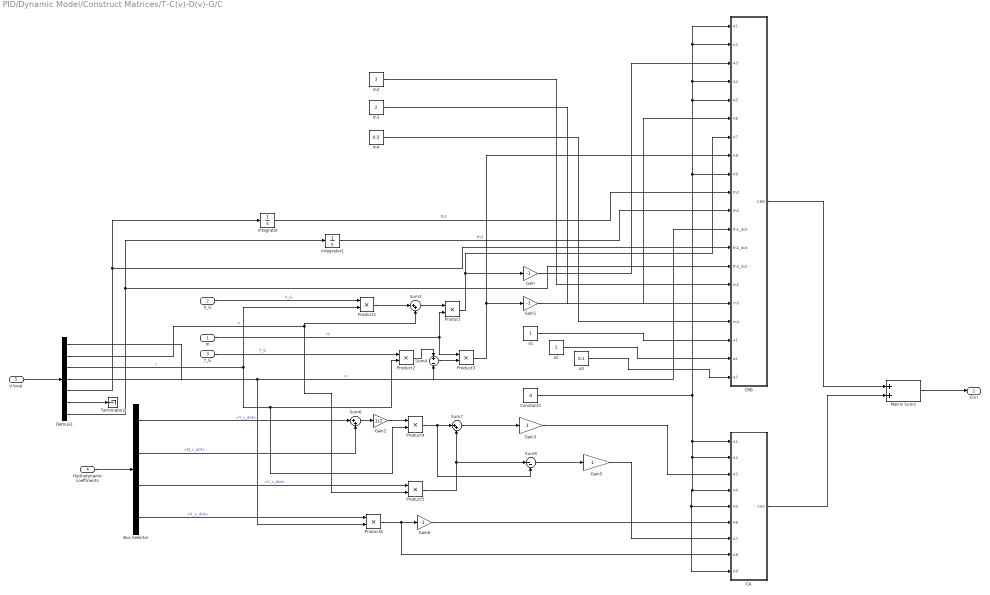
== system PID/Dynamic Model/Construct Matrices/T-C(v)-D(v)-G/C ==
  m : Inport
  X_G : Inport  Port=2
  Y_G : Inport  Port=3
  Hydrodynamic coefficients : Inport  Port=4
  V local : Inport  Port=5
  Bus Selector : BusSelector  OutputSignals=Y_r_dot,N_v_dot,Y_v_dot,X_u_dot
  CA : MATLAB Function  TreatAsAtomicUnit=on
  CRB : MATLAB Function  TreatAsAtomicUnit=on
  Constant3 : Constant  Value=0
  Demux1 : Demux  Outputs=7
  Gain : Gain  Gain=-1
  Gain1 : Gain  Gain=-1
  Gain2 : Gain  Gain=1/2
  Gain3 : Gain
  Gain5 : Gain
  Gain6 : Gain  Gain=-1
  Integrator : Integrator
  Integrator1 : Integrator
  Matrix Sum1 : Sum
  Product{,1..6} (7 alike) : Product
  Sum3 : Sum  Inputs=|++
  Sum4 : Sum  Inputs=+-
  Sum6 : Sum  Inputs=|++
  Sum7 : Sum  Inputs=|++
  Sum8 : Sum  Inputs=|--
  Terminator2 : Terminator
  a1 : Constant
  a2 : Constant
  a3 : Constant  Value=0.1
  m2 : Constant  Value=3
  m3 : Constant  Value=2
  m4 : Constant  Value=0.5
  C(v) : Outport
  wires:
  Hydrodynamic coefficients/1 -> Bus Selector/1
  Demux1/1 -> Product6/2, Sum4/2  "u"
  Gain3/1 -> CA/3(A3)
  CRB/1(CRB) -> Matrix Sum1/1
  Demux1/4 -> CRB/12(th1_dot)
  Product1/1 -> Sum3/1
  Gain6/1 -> CA/6(A6)
  Constant3/1 -> CRB/9(A9), CRB/2(A2), CRB/1(A1), CRB/4(A4), CRB/5(A5), CA/4(A4), CA/5(A5), CA/9(A9), CA/2(A2), CA/1(A1)
  Bus Selector/1 -> Sum6/1  "<Y_r_dot>"
  Product6/1 -> Gain6/1, CA/8(A8)
  Y_G/1 -> Product2/1  "Y_G"
  Sum3/1 -> Product/1
  Demux1/2 -> Product5/2, Sum3/2  "v"
  Bus Selector/2 -> Sum6/2  "<N_v_dot>"
  Demux1/7 -> Integrator1/1, CRB/14(th3_dot)
  Gain1/1 -> CRB/6(A6)
  Sum6/1 -> Gain2/1
  X_G/1 -> Product1/1  "X_G"
  Product5/1 -> Sum7/2, Sum8/1
  Demux1/6 -> Terminator2/1
  Gain2/1 -> Product4/1
  Bus Selector/4 -> Product6/1  "<X_u_dot>"
  Product3/1 -> Gain1/1, CRB/8(A8)
  m/1 -> Product/2, Product3/1  "m"
  Gain/1 -> CRB/3(A3)
  Demux1/5 -> CRB/13(th2_dot), Integrator/1
  Product/1 -> Gain/1, CRB/7(A7)
  Product2/1 -> Sum4/1
  Demux1/3 -> Product1/2, Product2/2, Product4/2  "r"
  Sum7/1 -> Gain3/1
  Sum8/1 -> Gain5/1
  Bus Selector/3 -> Product5/1  "<Y_v_dot>"
  CA/1(CA1) -> Matrix Sum1/2
  Matrix Sum1/1 -> C(v)/1
  Gain5/1 -> CA/7(A7)
  Sum4/1 -> Product3/2
  V local/1 -> Demux1/1
  Product4/1 -> Sum7/1, Sum8/2
  Integrator/1 -> CRB/10(th2)  "th2"
  Integrator1/1 -> CRB/11(th3)  "th3"
  m2/1 -> CRB/15(m2)
  m3/1 -> CRB/16(m3)
  m4/1 -> CRB/17(m4)
  a1/1 -> CRB/18(a1)
  a2/1 -> CRB/19(a2)
  a3/1 -> CRB/20(a3)

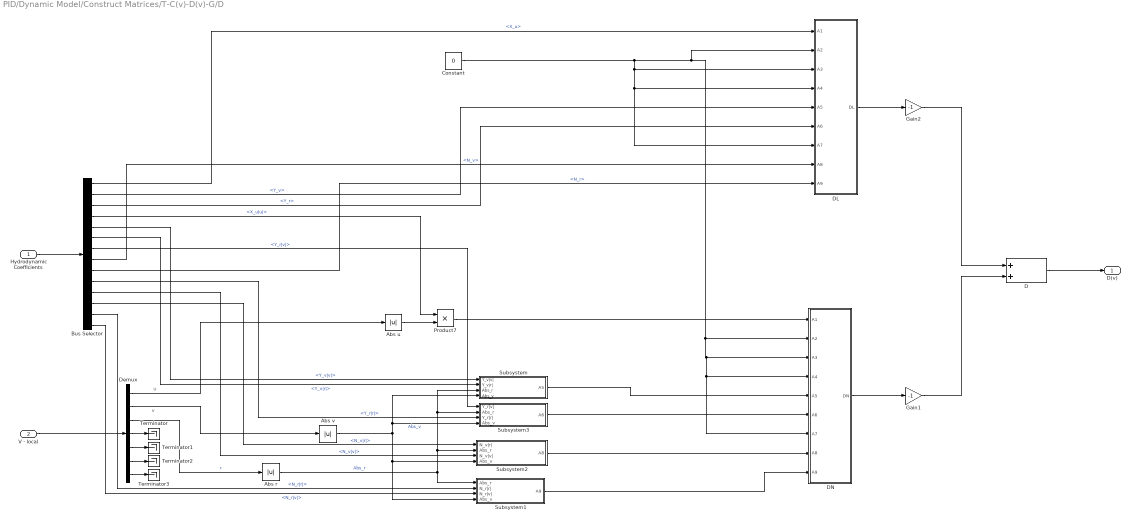
== system PID/Dynamic Model/Construct Matrices/T-C(v)-D(v)-G/D ==
  note: u
  note: v
  Hydrodynamic Coefficients : Inport
  V - local : Inport  Port=2
  Abs r : Abs  SaturateOnIntegerOverflow=off
  Abs u : Abs  SaturateOnIntegerOverflow=off
  Abs v : Abs  SaturateOnIntegerOverflow=off
  Bus Selector : BusSelector  OutputSignals=X_u,Y_v,Y_r,X_u|u|,Y_v|v|,Y_v|r|,Y_r|v|,N_v,N_r,Y_r|r|,N_v|v|,N_v|r|,N_r|r|,N_r|v|
  Constant : Constant  Value=0
  D : Sum
  DL : MATLAB Function  TreatAsAtomicUnit=on
  DN : MATLAB Function  TreatAsAtomicUnit=on
  Demux : Demux  Outputs=7
  Gain1 : Gain  Gain=-1
  Gain2 : Gain  Gain=-1
  Product7 : Product
  Subsystem : Subsystem
  Subsystem1 : Subsystem
  Subsystem2 : Subsystem
  Subsystem3 : Subsystem
  Terminator{,1..3} (4 alike) : Terminator
  D(v) : Outport
  wires:
  Demux/7 -> Terminator3/1
  Hydrodynamic Coefficients/1 -> Bus Selector/1
  Demux/6 -> Terminator2/1
  Demux/5 -> Terminator1/1
  Demux/1 -> Abs u/1
  Demux/4 -> Terminator/1
  Bus Selector/5 -> Subsystem/1("Y_v|v| ")  "<Y_v|v|>"
  Demux/2 -> Abs v/1
  Abs r/1 -> Subsystem/3(Abs_r), Subsystem3/2("Abs_r "), Subsystem2/2(Abs_r), Subsystem1/1(Abs_r)  "Abs_r"
  Gain1/1 -> D/2
  DL/1(DL) -> Gain2/1
  DN/1(DN) -> Gain1/1
  V - local/1 -> Demux/1
  Bus Selector/6 -> Subsystem/2(Y_v|r|)  "<Y_v|r|>"
  Demux/3 -> Abs r/1  "r"
  D/1 -> D(v)/1
  Gain2/1 -> D/1
  Subsystem2/1(A8) -> DN/8(A8)
  Bus Selector/4 -> Product7/1  "<X_u|u|>"
  Bus Selector/13 -> Subsystem1/2(N_r|r|)  "<N_r|r|>"
  Bus Selector/11 -> Subsystem2/3(N_v|v|)  "<N_v|v|>"
  Bus Selector/12 -> Subsystem2/1(N_v|r|)  "<N_v|r|>"
  Subsystem1/1(A9) -> DN/9(A9)
  Bus Selector/7 -> Subsystem3/1(Y_r|v|)  "<Y_r|v|>"
  Abs v/1 -> Subsystem/4("Abs_v "), Subsystem3/4(Abs_v), Subsystem1/4(Abs_v), Subsystem2/4(Abs_v)  "Abs_v"
  Constant/1 -> DL/2(A2), DN/2(A2), DN/3(A3), DN/4(A4), DN/7(A7), DL/4(A4), DL/7(A7), DL/3(A3)
  Bus Selector/14 -> Subsystem1/3(N_r|v|)  "<N_r|v|>"
  Abs u/1 -> Product7/2
  Subsystem/1(A5) -> DN/5(A5)
  Bus Selector/1 -> DL/1(A1)  "<X_u>"
  Subsystem3/1(A6) -> DN/6(A6)
  Product7/1 -> DN/1(A1)
  Bus Selector/10 -> Subsystem3/3(Y_r|r|)  "<Y_r|r|>"
  Bus Selector/9 -> DL/9(A9)  "<N_r>"
  Bus Selector/8 -> DL/8(A8)  "<N_v>"
  Bus Selector/3 -> DL/6(A6)  "<Y_r>"
  Bus Selector/2 -> DL/5(A5)  "<Y_v>"

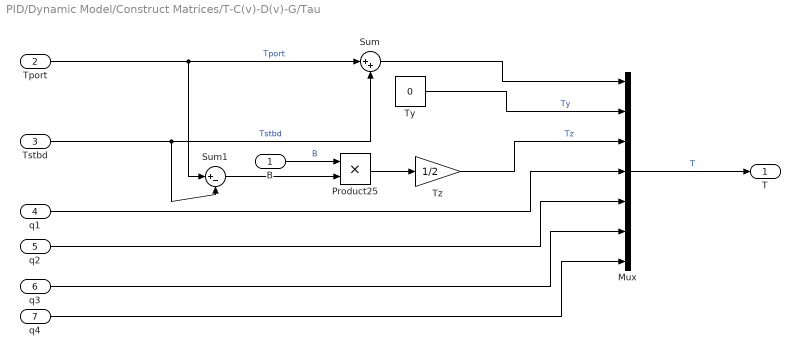
== system PID/Dynamic Model/Construct Matrices/T-C(v)-D(v)-G/Tau ==
  B : Inport
  Tport : Inport  Port=2
  Tstbd : Inport  Port=3
  q1 : Inport  Port=4
  q2 : Inport  Port=5
  q3 : Inport  Port=6
  q4 : Inport  Port=7
  Mux : Mux  Inputs=7
  Product25 : Product
  Sum : Sum  Inputs=|++
  Sum1 : Sum  Inputs=|+-
  Ty : Constant  Value=0
  Tz : Gain  Gain=1/2
  T : Outport  VectorParamsAs1DForOutWhenUnconnected=off
  wires:
  Tstbd/1 -> Sum/2, Sum1/2  "Tstbd"
  q3/1 -> Mux/6
  q2/1 -> Mux/5
  q1/1 -> Mux/4
  Tz/1 -> Mux/3  "Tz"
  Product25/1 -> Tz/1
  Sum1/1 -> Product25/2
  Mux/1 -> T/1  "T"
  Tport/1 -> Sum/1, Sum1/1  "Tport"
  Ty/1 -> Mux/2  "Ty"
  Sum/1 -> Mux/1
  q4/1 -> Mux/7
  B/1 -> Product25/1  "B"

== system PID/Dynamic Model/Construct Matrices/T-C(v)-D(v)-G/D/Subsystem ==
  "Y_v|v| " : Inport
  Y_v|r| : Inport  Port=2
  Abs_r : Inport  Port=3
  "Abs_v " : Inport  Port=4
  Product8 : Product
  Product9 : Product
  Sum10 : Sum  Inputs=|++
  A5 : Outport  VectorParamsAs1DForOutWhenUnconnected=off
  wires:
  Y_v|r|/1 -> Product9/1
  Abs_r/1 -> Product9/2
  Product9/1 -> Sum10/2
  "Y_v|v| "/1 -> Product8/1
  Product8/1 -> Sum10/1
  "Abs_v "/1 -> Product8/2
  Sum10/1 -> A5/1

== system PID/Dynamic Model/Construct Matrices/T-C(v)-D(v)-G/D/Subsystem1 ==
  Abs_r : Inport
  N_r|r| : Inport  Port=2
  N_r|v| : Inport  Port=3
  Abs_v : Inport  Port=4
  Product14 : Product
  Product15 : Product
  Sum13 : Sum  Inputs=|++
  A9 : Outport  VectorParamsAs1DForOutWhenUnconnected=off
  wires:
  Product15/1 -> Sum13/1
  Sum13/1 -> A9/1
  N_r|v|/1 -> Product14/1
  Product14/1 -> Sum13/2
  Abs_r/1 -> Product15/2
  N_r|r|/1 -> Product15/1
  Abs_v/1 -> Product14/2

== system PID/Dynamic Model/Construct Matrices/T-C(v)-D(v)-G/D/Subsystem2 ==
  N_v|r| : Inport
  Abs_r : Inport  Port=2
  N_v|v| : Inport  Port=3
  Abs_v : Inport  Port=4
  Product12 : Product
  Product13 : Product
  Sum12 : Sum  Inputs=|++
  A8 : Outport  VectorParamsAs1DForOutWhenUnconnected=off
  wires:
  Sum12/1 -> A8/1
  Product13/1 -> Sum12/1
  N_v|v|/1 -> Product12/1
  Product12/1 -> Sum12/2
  Abs_r/1 -> Product13/2
  Abs_v/1 -> Product12/2
  N_v|r|/1 -> Product13/1

== system PID/Dynamic Model/Construct Matrices/T-C(v)-D(v)-G/D/Subsystem3 ==
  Y_r|v| : Inport
  "Abs_r " : Inport  Port=2
  Y_r|r| : Inport  Port=3
  Abs_v : Inport  Port=4
  Product10 : Product
  Product11 : Product
  Sum11 : Sum  Inputs=|++
  A6 : Outport  VectorParamsAs1DForOutWhenUnconnected=off
  wires:
  Product11/1 -> Sum11/2
  Product10/1 -> Sum11/1
  Sum11/1 -> A6/1
  Y_r|v|/1 -> Product10/1
  "Abs_r "/1 -> Product11/2
  Y_r|r|/1 -> Product11/1
  Abs_v/1 -> Product10/2

== matlab function PID/MATLAB Function4 ==
  data: qw input; XYZ output; qx input; qy input; qz input
function XYZ = fcn(qw, qx, qy, qz)
quat = [qw qx qy qz];
XYZ = quat2eul(quat);

== matlab function PID/Wave Disturbance ==
  data: t input; tau_wave output
function tau_wave = WaveDisturbance3DOF(t)
%#codegen
% Simulink-compatible wave disturbance force/torque for 3DOF USV

% Constants
rho = 1000;      % Water density [kg/m^3]
g = 9.81;        % Gravity [m/s^2]
L = 4.29;        % Length overall [m]
B = 2.20;        % Beam [m]
T = 0.105;       % Draft [m]
x_G = 1.27;      % CG longitudinal [m]

% Wave heading (0 = surge, pi/2 = sway)
beta = pi/4;     % 45 degrees in radians

% Wave properties (3 harmonic components)
A = [0.3, 0.4, 0.2];                % Amplitudes [m]
lambda = [2.0, 3.0, 1.5];             % Wavelengths [m]
omega = sqrt(g * 2 * pi ./ lambda);   % Angular frequencies [rad/s]
phi = [0, pi/4, pi/2];                % Phases

% Initialize slope s_i(t)
s = zeros(1,3);
for i = 1:3
    s(i) = (A(i)/(2*pi*lambda(i))) * sin(omega(i)*t + phi(i));
end

% Compute wave-induced forces
X_wave = sum(rho * g * B * L * T * cos(beta) * s);
Y_wave = -sum(rho * g * B * L * T * sin(beta) * s);
N_wave = sum((1/24) * rho * g * B * L * (L^2 - B^2) * sin(2*beta) * s.^2);

% Output vector
tau_wave = [X_wave; Y_wave; N_wave; 0; 0; 0; 0];

== matlab function PID/Controller/Subsystem5/MATLAB Function ==
  data: A1 input; A2 input; A3 input; A4 input; A5 input; A6 input; A7 input; A8 input; A9 input; J1 output
function J1 = fcn(A1, A2, A3, A4, A5, A6, A7, A8, A9)

J1 = [A1,A2,A3,0,0,0,0;
    A4,A5,A6,0,0,0,0;
    A7,A8,A9,0,0,0,0;
    0,0,0,1,0,0,0;
    0,0,0,0,1,0,0;
    0,0,0,0,0,1,0;
    0,0,0,0,0,0,1;];

== matlab function PID/Dynamic Model/Construct Matrices/M/MATLAB Function ==
  data: A1 input; A2 input; A3 input; A4 input; A5 input; A6 input; A7 input; A8 input; A9 input; M output; m1 input; m2 input; m3 input; m4 input; a1 input; a2 input; a3 input; th2 input; th3 input
function M = fcn(A1, A2, A3, A4, A5, A6, A7, A8, A9, m1, m2, m3, m4, a1, a2, a3, th2, th3)

% Define the expressions for M
m11 = (a1^2*m1)/4 + a1^2*m2 + a1^2*m3 + (a2^2*m2)/4 + a1^2*m4 + a2^2*m3 + a2^2*m4 + a3^2*m4 + 2*a1*a3*m4*cos(th2 + th3) + a1*a2*m2*cos(th2) + 2*a1*a2*m3*cos(th2) + 2*a1*a2*m4*cos(th2) + 2*a2*a3*m4*cos(th3);
m12 = (a2^2*m2)/4 + a2^2*m3 + a2^2*m4 + a3^2*m4 + a1*a3*m4*cos(th2 + th3) + (a1*a2*m2*cos(th2))/2 + a1*a2*m3*cos(th2) + a1*a2*m4*cos(th2) + 2*a2*a3*m4*cos(th3);
m13 = 0;
m14 = a3^2*m4 + a1*a3*m4*cos(th2 + th3) + a2*a3*m4*cos(th3);
m21 = (a2^2*m2)/4 + a2^2*m3 + a2^2*m4 + a3^2*m4 + a1*a3*m4*cos(th2 + th3) + (a1*a2*m2*cos(th2))/2 + a1*a2*m3*cos(th2) + a1*a2*m4*cos(th2) + 2*a2*a3*m4*cos(th3);
m22 = (a2^2*m2)/4 + a2^2*m3 + a2^2*m4 + a3^2*m4 + 2*a2*a3*m4*cos(th3);
m23 = 0;
m24 = m4*a3^2 + a2*m4*cos(th3)*a3;
m31 = 0;
m32 = 0;
m33 = (m3 + 4*m4)/4;
m34 = 0;
m41 = a3^2*m4 + a3*m4*a1*cos(th2 + th3) + a3*m4*a2*cos(th3);
m42 = a3^2*m4 + a3*m4*a2*cos(th3);
m43 = 0;
m44 = a3^2*m4;

M = [A1,A2,A3,0,0,0,0;
    A4,A5,A6,0,0,0,0;
    A7,A8,A9,0,0,0,0;
    0,0,0,m11,m12,m13,m14;
    0,0,0,m21,m22,m23,m24;
    0,0,0,m31,m32,m33,m34;
    0,0,0,m41,m42,m43,m44];

== matlab function PID/Dynamic Model/Construct Matrices/M^-1 ==
  data: u input; y output
function y = fcn(u)
y = inv(u);

== matlab function PID/Dynamic Model/Construct Matrices/T-C(v)-D(v)-G/C/CA ==
  data: A1 input; A2 input; A3 input; A4 input; A5 input; A6 input; A7 input; A8 input; A9 input; CA1 output
function CA1 = fcn(A1, A2, A3, A4, A5, A6, A7, A8, A9)

CA1 = [A1,A2,A3,0,0,0,0;
    A4,A5,A6,0,0,0,0;
    A7,A8,A9,0,0,0,0;
    0,0,0,0,0,0,0;
    0,0,0,0,0,0,0;
    0,0,0,0,0,0,0;
    0,0,0,0,0,0,0;];

== matlab function PID/Dynamic Model/Construct Matrices/T-C(v)-D(v)-G/C/CRB ==
  data: A1 input; A2 input; A3 input; A4 input; A5 input; A6 input; A7 input; A8 input; A9 input; CRB output; th2 input; th3 input; th1_dot input; th2_dot input; th3_dot input; m2 input; m3 input; m4 input; a1 input; a2 input; a3 input
function CRB = fcn(A1, A2, A3, A4, A5, A6, A7, A8, A9, th2, th3, th1_dot, th2_dot, th3_dot, m2, m3, m4, a1, a2, a3)

% Define the expressions for C
c11 = -2*a1*a3*m4*sin(th2 + th3) + th2_dot + th3_dot - a1*a2*m2*sin(th2) - 2*a1*a2*m3*sin(th2) - 2*a1*a2*m4*sin(th2) - 2*a2*a3*m4*sin(th3);
c12 = -a1*a3*m4*sin(th2 + th3) + th2_dot + th3_dot - (a1*a2*m2*sin(th2))/2 - a1*a2*m3*sin(th2) - a1*a2*m4*sin(th2) - 2*a2*a3*m4*sin(th3);
c13 = 0;
c14 = -a1*a3*m4*sin(th2 + th3) + th2_dot + th3_dot - a2*a3*m4*sin(th3);
c21 = ((a1*(a2*m2*sin(th2) + 2*a2*m3*sin(th2) + 2*a2*m4*sin(th2) + 2*a3*m4*sin(th2 + th3)))/2)*th1_dot + - a1*a3*m4*sin(th2 + th3) - (a1*a2*m2*sin(th2))/2 - a1*a2*m3*sin(th2) - a1*a2*m4*sin(th2) - 2*a2*a3*m4*sin(th3);
c22 = ((a1*(a2*m2*sin(th2) + 2*a2*m3*sin(th2) + 2*a2*m4*sin(th2) + 2*a3*m4*sin(th2 + th3)))/2 + 1)*th1_dot - 2*a2*a3*m4*sin(th3);
c23 = 0;
c24 = (a1*a3*m4*sin(th2 + th3) + 1)*th1_dot - a2*a3*m4*sin(th3);
c31 = 0;
c32 = 0;
c33 = 0;
c34 = 0;
c41 = a2*sin(th3)*th1_dot - a1*a3*m4*sin(th2 + th3) - a2*a3*m4*sin(th3);
c42 = (a3*m4*(a1*sin(th2 + th3) + a2*sin(th3)) + a2*a3*m4*sin(th3) + 1)*th1_dot + a2*a3*m4*sin(th3)*th2_dot -a2*a3*m4*sin(th3);
c43 = 0;
c44 = a2*a3*m4*sin(th3)*th2_dot + (a3*m4*(a1*sin(th2 + th3) + a2*sin(th3)) + 1)*th1_dot;

CRB = [A1,A2,A3,0,0,0,0;
    A4,A5,A6,0,0,0,0;
    A7,A8,A9,0,0,0,0;
    0,0,0,c11,c12,c13,c14;
    0,0,0,c21,c22,c23,c24;
    0,0,0,c31,c32,c33,c34;
    0,0,0,c41,c42,c43,c44];

== matlab function PID/Dynamic Model/Construct Matrices/T-C(v)-D(v)-G/D/DL ==
  data: A1 input; A2 input; A3 input; A4 input; A5 input; A6 input; A7 input; A8 input; A9 input; DL output
function DL = fcn(A1, A2, A3, A4, A5, A6, A7, A8, A9)

DL = [A1,A2,A3,0,0,0,0;
    A4,A5,A6,0,0,0,0;
    A7,A8,A9,0,0,0,0;
    0,0,0,1,0,0,0;
    0,0,0,0,1,0,0;
    0,0,0,0,0,1,0;
    0,0,0,0,0,0,1;];

== matlab function PID/Dynamic Model/Construct Matrices/T-C(v)-D(v)-G/D/DN ==
  data: A1 input; A2 input; A3 input; A4 input; A5 input; A6 input; A7 input; A8 input; A9 input; DN output
function DN = fcn(A1, A2, A3, A4, A5, A6, A7, A8, A9)

DN = [A1,A2,A3,0,0,0,0;
    A4,A5,A6,0,0,0,0;
    A7,A8,A9,0,0,0,0;
    0,0,0,0,0,0,0;
    0,0,0,0,0,0,0;
    0,0,0,0,0,0,0;
    0,0,0,0,0,0,0];

== matlab function PID/Dynamic Model/Construct Matrices/T-C(v)-D(v)-G/G ==
  data: m3 input; G output; m4 input; g input
function G = fcn(m3, m4, g)

% Define the expressions for G
g1 = 0
g2 = 0
g3 = g*(m3 + m4)
g4 = 0

G = [0;0;0;g1;g2;g3;g4];

== matlab function PID/MATLAB Function1 ==
  data: th1 input; T output; th2 input; d input; th3 input; h input; L1 input; L2 input; L3 input
function T = fcn(th1, th2, d,th3, h, L1, L2, L3)
T = [cos(th1 + th2 + th3), -sin(th1 + th2 + th3), 0, L1*cos(th1) + L2*cos(th1 + th2) + L3*cos(th1 + th2 + th3);
    sin(th1 + th2 + th3), cos(th1 + th2 + th3), 0, L1*sin(th1) + L2*sin(th1 + th2) + L3*sin(th1 + th2 + th3);
    0, 0, 1, h-d;
    0,0,0,1];

== matlab function PID/Controller/MATLAB Function ==
  data: u input; y output
function y = fcn(u)

y = inv(u);

== matlab function PID/MATLAB Function2 ==
  data: Px input; Py input; Pz input; L1 input; L2 input; h input; q1 output; q2 output; q3 output; q4 output
function [q1, q2, q3, q4] = fcn(Px,Py,Pz,L1,L2,h)

c2 = (Px^2 + Py^2 - L1^2 - L2^2)/(2*L1*L2);

q2 = acos((Px^2 + Py^2 - L1^2 - L2^2)/(2*L1*L2));
q1 = atan((-L2*sin(q2)*Px + (L1 + L2*cos(q2))*Py)/(L2*sin(q2)*Py + (L1 + L2*cos(q2))*Px));
q3 = Pz-h;
a = sin(q1 + q2);
b = cos(q1 + q2);
q4 = atan(-a/b)-q1-q2;
